simulink model "DC_2016"  (R2016b)
settings: Solver=FixedStepAuto  StartTime=0.0  StopTime=t_max  FixedStep=timestep  RelTol=1e-3
values from neighbouring files (symbols this model uses):
  den = [J*La (Ra*J+B*La) (Ra*B+Kb^2) 0]    [DC_MOTOR_analisys.m]
  K = -sym2poly(routh(transfer))    [DC_MOTOR_analisys.m]
  num = Kb    (= 1.2)    [DC_MOTOR_analisys.m]
  step_v = 1    [DC_MOTOR_analisys.m]
settings Model: Creator=mluser  LastModifiedBy=Gabriel
settings DataIOCC: ReturnWorkspaceOutputs=on
settings DebuggingCC: UnconnectedInputMsg=none  UnconnectedOutputMsg=none  UnconnectedLineMsg=none
settings ModelReferenceCC: EnableRefExpFcnMdlSchedulingChecks=off
settings SFSimCC: SimUseLocalCustomCode=on
settings RTWCC: RTWUseLocalCustomCode=on

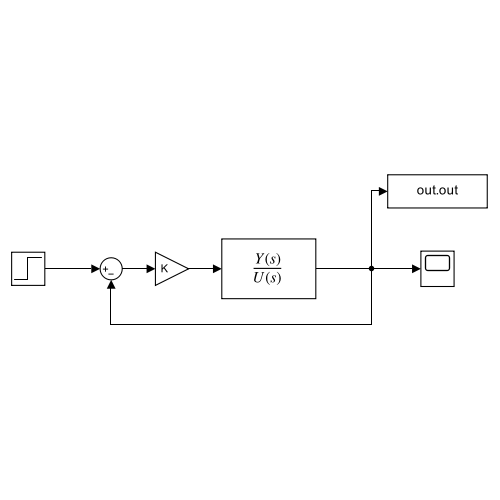
[thumbnail: Simulink's stored preview of the top-level diagram]
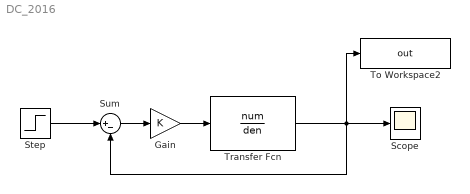
== system DC_2016 ==
  Gain : Gain  Gain=K
  Scope : Scope
  Step : Step  Time=0  After=step_v  SampleTime=0
  Sum : Sum  Inputs=|+-
  To Workspace2 : ToWorkspace  VariableName=out  SampleTime=-1
  Transfer Fcn : TransferFcn  Numerator=num  Denominator=den
  wires:
  Transfer Fcn/1 -> Sum/2, To Workspace2/1, Scope/1
  Step/1 -> Sum/1
  Gain/1 -> Transfer Fcn/1
  Sum/1 -> Gain/1
